simulink model "PMSM_FOC_Tractio"  (R2019b)
settings: Solver=FixedStepAuto  StartTime=0.0  StopTime=10  RelTol=1e-3
model workspace (MAT data in the model file):
  wc : Simulink.Parameter (value not decoded)
values from neighbouring files (symbols this model uses):
  Cosine_table = 1.0 0.99999529 0.99999058 0.99998587 0.99998116 0.99996704 0.99995291 0.99993885 0.99992472 0.99990118 0.99987763 0.99985409 0.9998306 0.99979764 0.99976468 0.99973178 0.99969882 0.99965644 0.99961412 0.99957174 0.99952942 0.99947762 0.99942589 0.99937415 0.99932235 0.9992612 0.99920005 0.99913889 0.99907768 0.99900717 0.99893659 0.99886602 0.99879545 0.99871546 0.99863547 0.99855554 0.99847555 0.    [Hall_HFI_FOC_Data.sldd]
  Flux = 0.00529276    [Hall_HFI_FOC_Data.sldd]
  MTPA_id_table = 0.22889 0.23462678 0.23770036 0.2381243 0.23591207 0.23107713 0.2236329 0.21359272 0.20096992 0.18577772 0.16802935 0.14773798 0.12491672 0.099578641 0.071736768 0.041404068 0.0085934745 -0.026682133 -0.064409919 -0.10457709 -0.14717092 -0.1921787 -0.2395878 -0.28938559 -0.34155953 -0.39609709 -0.45298585 -0.51221335 -0.57376724 -0.63763517 -0.70380485 -0.77226412 -0.84300071 -0.91600245 -0.991257    [Hall_HFI_FOC_Data.sldd]
  MTPA_iq_table = -1.0417 -0.16083497 0.71926296 1.5985928 2.4771533 3.3549435 4.2319627 5.1082091 5.9836826 6.8583813 7.732305 8.6054525 9.4778223 10.349415 11.220228 12.090261 12.959513 13.827983 14.69567 15.562573 16.428694 17.294027 18.158575 19.022335 19.885307 20.747492 21.608887 22.469492 23.329306 24.188328 25.046556 25.903992 26.760633 27.616482 28.471533 29.325788 30.179247 31.031908 31.883772 32.734837 3    [Hall_HFI_FOC_Data.sldd]
  MTPA_Te_Max = 800.0    [Hall_HFI_FOC_Data.sldd]
  MTPA_Te_Min = 0.0    [Hall_HFI_FOC_Data.sldd]
  Sine_table = 0.0 0.0015339879 0.0030679768 0.0046019657 0.0061359555 0.0076698866 0.0092038177 0.010737749 0.012271681 0.013805497 0.015339312 0.016873131 0.018406944 0.019940587 0.021474229 0.023007872 0.024541514 0.026074925 0.027608337 0.029141748 0.03067516 0.032208283 0.033741407 0.035274528 0.036807653 0.038340431 0.039873205 0.04140598 0.042938754 0.04447113 0.046003502 0.047535874 0.049068246 0.0506001    [Hall_HFI_FOC_Data.sldd]
undefined symbols (not defined in the file or in its folder): CL_Param, ctrlParamsPI, DiscIntNeverNeededParam, Flux_weak, HFI, inverter, magnitude, OPL_Param, pmsm, sigbuilder_block, SMO, SVPWM
libraries: powerlib x22, fl_lib x18, simulink x7, nesl_utility x7, powerlib_meascontrol x3, dspstat3 x3, powerlib_extras x1, ee_lib x1
(part 2 of 4)

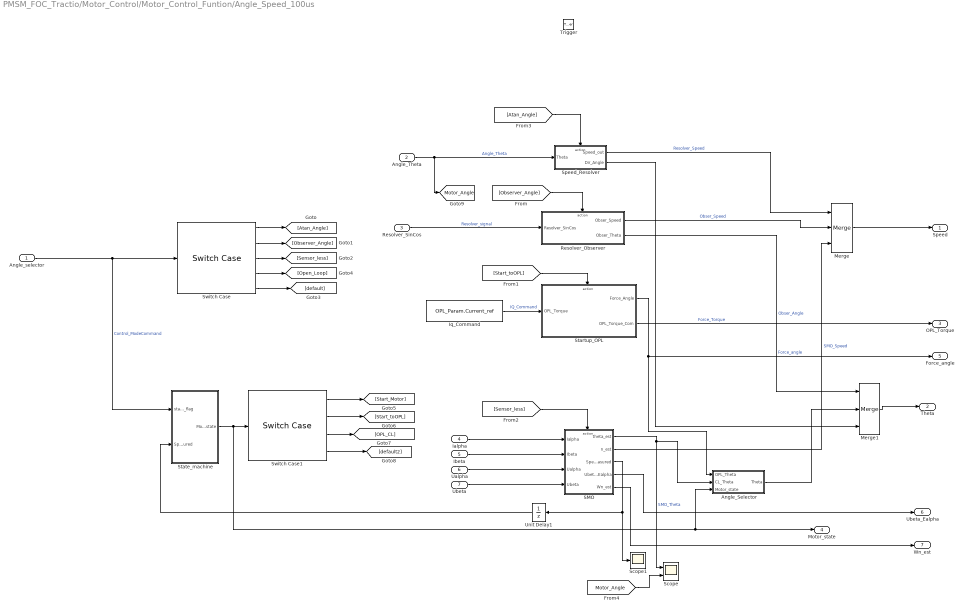
== system PMSM_FOC_Tractio/Motor_Control/Motor_Control_Funtion/Angle_Speed_100us ==
  Angle_selector : Inport
  Angle_Theta : Inport  Port=2  OutMin=0  OutMax=2*pi
  Resolver_SinCos : Inport  Port=3  OutMin=0  OutMax=2*pi
  Ialpha : Inport  Port=4
  Ibeta : Inport  Port=5
  Ualpha : Inport  Port=6
  Ubeta : Inport  Port=7
  Trigger : TriggerPort  TriggerType=function-call  VariantControl=Variant  SampleTimeType=periodic  SampleTime=-1  PortDimensions=1
  Angle_Selector : Subsystem  TreatAsAtomicUnit=on
      settings: RTWSystemCode=Nonreusable function  RTWFcnNameOpts=Use subsystem name
  Iq_Command : Constant  Value=OPL_Param.Current_ref  SampleTime=-1
  Merge : Merge  Inputs=3
  Merge1 : Merge  Inputs=3
  Resolver_Observer : Subsystem
      settings: RTWSystemCode=Nonreusable function  RTWFcnNameOpts=Use subsystem name
  SMO : Subsystem  TreatAsAtomicUnit=on
      settings: RTWSystemCode=Nonreusable function  RTWFcnNameOpts=Use subsystem name
  Scope : Scope  NumInputPorts=2
  Scope1 : Scope
  Speed_Resolver : Subsystem  TreatAsAtomicUnit=on
      settings: RTWSystemCode=Nonreusable function  RTWFcnNameOpts=Use subsystem name
  Startup_OPL : Subsystem  TreatAsAtomicUnit=on  SystemSampleTime=inverter.Ts
      settings: RTWSystemCode=Nonreusable function  RTWFcnNameOpts=Use subsystem name
  State_machine : Stateflow chart  BlockKeywords=__PRM__SERIALIZED__DATA__:Stateflow Chart,Stateflow Diagram  TreatAsAtomicUnit=on
      settings: RTWSystemCode=Nonreusable function  RTWFcnNameOpts=Use subsystem name
  Switch Case : SwitchCase  CaseConditions={1,2,3,4}
  Switch Case1 : SwitchCase  CaseConditions={1,2,3}
  Unit Delay1 : UnitDelay  SampleTime=-1  HasFrameUpgradeWarning=on
  Speed : Outport
  Theta : Outport  Port=2
  OPL_Torque : Outport  Port=3
  Motor_state : Outport  Port=4
  Force_angle : Outport  Port=5
  Ubeta_Ealpha : Outport  Port=6
  Wn_est : Outport  Port=7
  tag scope: Motor_Angle=global
  wires:
  [Start_toOPL] -> Startup_OPL/Action
  [Sensor_less] -> SMO/Action
  Resolver_SinCos/1 -> Resolver_Observer/1(Resolver_SinCos)  "Resolver_signal"
  [Observer_Angle] -> Resolver_Observer/Action
  Iq_Command/1 -> Startup_OPL/1(OPL_Torque)  "IQ_Command"
  Resolver_Observer/2(Obser_Theta) -> Merge1/1  "Obser_Angle"
  Ialpha/1 -> SMO/1(Ialpha)
  Ibeta/1 -> SMO/2(Ibeta)
  Ualpha/1 -> SMO/3(Ualpha)
  Ubeta/1 -> SMO/4(Ubeta)
  Merge/1 -> Speed/1
  Merge1/1 -> Theta/1
  Angle_selector/1 -> State_machine/1(start_flag), Switch Case/1  "Control_ModeCommand"
  Switch Case/5 -> [default]
  Switch Case/3 -> [Sensor_less]
  Switch Case/1 -> [Atan_Angle]
  Switch Case/4 -> [Open_Loop]
  Switch Case/2 -> [Observer_Angle]
  Speed_Resolver/1(Speed_out) -> Merge/1  "Resolver_Speed"
  Angle_Theta/1 -> [Motor_Angle], Speed_Resolver/1(Theta)  "Angle_Theta"
  [Atan_Angle] -> Speed_Resolver/Action
  SMO/2(n_est) -> Merge/3  "SMO_Speed"
  Resolver_Observer/1(Obser_Speed) -> Merge/2  "Obser_Speed"
  Startup_OPL/2(OPL_Torque_Com) -> OPL_Torque/1  "Force_Torque"
  Speed_Resolver/2(Dir_Angle) -> Merge1/3
  Switch Case1/3 -> [OPL_CL]
  Switch Case1/2 -> [Start_toOPL]
  Switch Case1/1 -> [Start_Motor]
  Switch Case1/4 -> [default2]
  State_machine/1(Motor_state) -> Angle_Selector/3(Motor_state), Motor_state/1, Switch Case1/1
  Unit Delay1/1 -> State_machine/2(Speed_Measured)
  SMO/1(theta_est) -> Scope/1, Angle_Selector/2(CL_Theta)  "SMO_Theta"
  Startup_OPL/1(Force_Angle) -> Angle_Selector/1(OPL_Theta), Force_angle/1  "Force_angle"
  Angle_Selector/1(Theta) -> Merge1/2
  [Motor_Angle] -> Scope/2
  SMO/3(Speed_Measured) -> Unit Delay1/1, Scope1/1
  SMO/4(Ubeta_Ealpha) -> Ubeta_Ealpha/1
  SMO/5(Wn_est) -> Wn_est/1

== system PMSM_FOC_Tractio/Motor_Control/Motor_Control_Funtion/Control_Command_2ms ==
  Control_Mode : Inport
  Speed_target : Inport  Port=2
  Speed_Mesured : Inport  Port=3  OutMin=0  OutMax=2*pi
  HFI_State : Inport  Port=4
  Trigger : TriggerPort  TriggerType=function-call  VariantControl=Variant  SampleTimeType=periodic  SampleTime=-1  PortDimensions=1
  IQ_Command : Constant  Value=CL_Param.Current_IQref  OutDataTypeStr=single  SampleTime=-1
  Merge : Merge
  Speed_PI : Subsystem  TreatAsAtomicUnit=on  SystemSampleTime=inverter.Ts
      settings: RTWSystemCode=Nonreusable function
  Switch Case : SwitchCase  CaseConditions={1,2}
  Switch Case Action Subsystem : Subsystem  TreatAsAtomicUnit=on
      settings: RTWSystemCode=Nonreusable function
  Te_ref : Outport
  wires:
  Switch Case Action Subsystem/1(Iq_out) -> Merge/2
  IQ_Command/1 -> Switch Case Action Subsystem/1(Iq_in)  "IQ_Command"
  Switch Case/3 -> [default]
  [Torque_Mode] -> Switch Case Action Subsystem/Action
  Switch Case/2 -> [Torque_Mode]
  Switch Case/1 -> [Speed_Mode]
  Control_Mode/1 -> Switch Case/1  "Control_ModeCommand"
  [Speed_Mode] -> Speed_PI/Action
  Speed_PI/1(Iq_ref) -> Merge/1  "Iq_ref"
  Merge/1 -> Te_ref/1
  Speed_target/1 -> Speed_PI/1(Speed_Command)  "Speed_target"
  Speed_Mesured/1 -> Speed_PI/2(Speed_Measured)  "Speed_Measured"
  HFI_State/1 -> Speed_PI/3(HFI_State)  "Control_ModeCommand"

== system PMSM_FOC_Tractio/Motor_Control/Motor_Control_Funtion/FOC_Control_100us ==
  Phase_CurrentABC : Inport  PortDimensions=3
  Angle_Theta : Inport  Port=2  OutMin=0  OutMax=2*pi
  Te_ref : Inport  Port=3
  Motor_state : Inport  Port=4
  OPL_Iq : Inport  Port=5
  Trigger : TriggerPort  TriggerType=function-call  VariantControl=Variant  SampleTimeType=periodic  SampleTime=-1  PortDimensions=1
  FOC : Subsystem  TreatAsAtomicUnit=on
      settings: RTWSystemCode=Nonreusable function  RTWFcnNameOpts=Use subsystem name
  Iq_selector : Subsystem  TreatAsAtomicUnit=on
      settings: RTWSystemCode=Nonreusable function  RTWFcnNameOpts=Use subsystem name
  MTPA : Subsystem  TreatAsAtomicUnit=on
      settings: RTWSystemCode=Nonreusable function  RTWFcnNameOpts=Use subsystem name
  Ta : Outport
  Tb : Outport  Port=2
  Tc : Outport  Port=3
  Ialpha : Outport  Port=4
  Ibeta : Outport  Port=5
  Valpha : Outport  Port=6
  Vbeta : Outport  Port=7
  Id : Outport  Port=8
  Iq : Outport  Port=9
  HFI_Theta : Outport  Port=10
  RUN_State : Outport  Port=11
  HFI_Speed : Outport  Port=12
  wires:
  FOC/1(Ta) -> Ta/1  "Ta"
  FOC/2(Tb) -> Tb/1  "Tb"
  FOC/3(Tc) -> Tc/1  "Tc"
  Angle_Theta/1 -> FOC/3(Angle_Theta)  "Angle_Theta"
  FOC/4(Ialpha) -> Ialpha/1  "Ialpha"
  FOC/5(Ibeta) -> Ibeta/1  "Ibeta"
  FOC/6(Valpha) -> Valpha/1  "V_alpha"
  FOC/7(Vbeta) -> Vbeta/1  "V_beta"
  FOC/8(Id) -> Id/1  "Id_measured"
  FOC/9(Iq) -> Iq/1  "Iq_measured"
  Phase_CurrentABC/1 -> FOC/4(Phase_CurrentABC)  "Phase_CurrentABC"
  FOC/11(HFI_Theta) -> HFI_Theta/1  "HFI_Theta"
  FOC/10(RUN_State) -> RUN_State/1
  FOC/12(HFI_Speed) -> HFI_Speed/1
  MTPA/1(Id_ref) -> FOC/1(Id_target)  "Id_ref"
  MTPA/2(Iq_ref) -> Iq_selector/2(PI_IQ)  "Iq_ref"
  Iq_selector/1(Iq_ref) -> FOC/2(Iq_target)
  Te_ref/1 -> MTPA/1(Te_ref)
  Motor_state/1 -> Iq_selector/1(Motor_state)
  OPL_Iq/1 -> Iq_selector/3(OPL_IQ)

== system PMSM_FOC_Tractio/PMSM/Resolver/Meas Vxy ==
  Electrical Reference{1..4} (4 alike) : fl_lib/Electrical/Electrical Elements/Electrical Reference
  PS-Simulink Converter : nesl_utility/PS-Simulink Converter  PhysicalDomain=network_engine_domain  SubClassName=ps_output  LeftPortType=input  RightPortType=output  PseudoPeriodic=off  Frequencies=[]  Unit=1  AffineConversion=off
  PS-Simulink Converter1 : nesl_utility/PS-Simulink Converter  PhysicalDomain=network_engine_domain  SubClassName=ps_output  LeftPortType=input  RightPortType=output  PseudoPeriodic=off  Frequencies=[]  Unit=1  AffineConversion=off
  Resistor : fl_lib/Electrical/Electrical Elements/Resistor  R=1e3 Ohm  i_specify=off  i_priority=None  i=0 A  i_nominal_specify=off  i_nominal_unit=A  i_nominal_value=1  v_specify=off  v_priority=None  v=0 V  v_nominal_specify=off  v_nominal_unit=V  v_nominal_value=1
  Resistor1 : fl_lib/Electrical/Electrical Elements/Resistor  R=1e3 Ohm  i_specify=off  i_priority=None  i=0 A  i_nominal_specify=off  i_nominal_unit=A  i_nominal_value=1  v_specify=off  v_priority=None  v=0 V  v_nominal_specify=off  v_nominal_unit=V  v_nominal_value=1
  VS1 : fl_lib/Electrical/Electrical Sensors/Voltage Sensor
  VS2 : fl_lib/Electrical/Electrical Sensors/Voltage Sensor
  x1 : PMIOPort  Side=Left
  x2 : PMIOPort  Port=2  Side=Left
  y1 : PMIOPort  Port=3  Side=Left
  y2 : PMIOPort  Port=4  Side=Left
  Vx : Outport  VectorParamsAs1DForOutWhenUnconnected=off
  Vy : Outport  Port=2  VectorParamsAs1DForOutWhenUnconnected=off
  wires:
  PS-Simulink Converter1/1 -> Vy/1
  PS-Simulink Converter/1 -> Vx/1
  connections:
  VS1/RConn1 -- PS-Simulink Converter/LConn1
  Resistor/RConn1 -- x2/RConn1 -- Electrical Reference2/LConn1
  Electrical Reference1/LConn1 -- VS1/RConn2
  y2/RConn1 -- Electrical Reference4/LConn1 -- Resistor1/RConn1
  VS2/LConn1 -- y1/RConn1 -- Resistor1/LConn1
  Electrical Reference3/LConn1 -- VS2/RConn2
  VS2/RConn1 -- PS-Simulink Converter1/LConn1
  Resistor/LConn1 -- x1/RConn1 -- VS1/LConn1

== system PMSM_FOC_Tractio/PMSM/Resolver/Vp ==
  Electrical Reference1 : fl_lib/Electrical/Electrical Elements/Electrical Reference
  PS-Simulink Converter2 : nesl_utility/PS-Simulink Converter  PhysicalDomain=network_engine_domain  SubClassName=ps_output  LeftPortType=input  RightPortType=output  PseudoPeriodic=off  Frequencies=[]  Unit=1  AffineConversion=off
  VS1 : fl_lib/Electrical/Electrical Sensors/Voltage Sensor
  Vp1 : fl_lib/Electrical/Electrical Sources/AC Voltage Source  amp=5 V  shift=0 rad  frequency=1e4 Hz  omega=0 rad/s
  p1 : PMIOPort  Side=Right
  p2 : PMIOPort  Port=2  Side=Right
  Vp : Outport  VectorParamsAs1DForOutWhenUnconnected=off
  wires:
  PS-Simulink Converter2/1 -> Vp/1
  connections:
  VS1/RConn1 -- PS-Simulink Converter2/LConn1
  Electrical Reference1/LConn1 -- p2/RConn1 -- VS1/RConn2 -- Vp1/RConn1
  VS1/LConn1 -- Vp1/LConn1 -- p1/RConn1

== system PMSM_FOC_Tractio/PMSM/Resolver_SinCos/If Action Subsystem ==
  In1 : Inport
  Action Port : ActionPort  ActionPortLabel=if(u1 == 1)
  Out1 : Outport
  wires:
  In1/1 -> Out1/1

== system PMSM_FOC_Tractio/PMSM/Resolver_SinCos/If Action Subsystem1 ==
  In1 : Inport
  Action Port : ActionPort  ActionPortLabel=else
  Gain : Gain  Gain=-1
  Out1 : Outport
  wires:
  In1/1 -> Gain/1
  Gain/1 -> Out1/1

== system PMSM_FOC_Tractio/PMSM/Resolver_SinCos/If Action Subsystem2 ==
  In1 : Inport
  Action Port : ActionPort  ActionPortLabel=if(u1 == 1)
  Out1 : Outport
  wires:
  In1/1 -> Out1/1

== system PMSM_FOC_Tractio/PMSM/Resolver_SinCos/If Action Subsystem3 ==
  In1 : Inport
  Action Port : ActionPort  ActionPortLabel=else
  Gain : Gain  Gain=-1
  Out1 : Outport
  wires:
  In1/1 -> Gain/1
  Gain/1 -> Out1/1

== system PMSM_FOC_Tractio/PMSM/Resolver_SinCos/Subsystem ==
  In1 : Inport
  Trigger : TriggerPort  VariantControl=Variant  SampleTimeType=periodic  SampleTime=-1  PortDimensions=1
  Out1 : Outport
  wires:
  In1/1 -> Out1/1

== system PMSM_FOC_Tractio/PMSM/Resolver_SinCos/Subsystem1 ==
  In1 : Inport
  Trigger : TriggerPort  VariantControl=Variant  SampleTimeType=periodic  SampleTime=-1  PortDimensions=1
  Out1 : Outport
  wires:
  In1/1 -> Out1/1

== system PMSM_FOC_Tractio/PMSM/Resolver_SinCos/Subsystem2 ==
  Trigger : TriggerPort  VariantControl=Variant  SampleTimeType=periodic  SampleTime=-1  PortDimensions=1
  Add : Sum
  Constant : Constant
  Constant1 : Constant  Value=2
  Memory : Memory  InheritSampleTime=on
  Mod : Math  Operator=mod  SignedPower=off  SaturateOnIntegerOverflow=on
  Out1 : Outport
  wires:
  Add/1 -> Mod/1, Memory/1
  Constant/1 -> Add/1
  Memory/1 -> Add/2
  Mod/1 -> Out1/1  "Theta"
  Constant1/1 -> Mod/2

== system PMSM_FOC_Tractio/PMSM/Resolver_SinCos/Subsystem3 ==
  Trigger : TriggerPort  VariantControl=Variant  SampleTimeType=periodic  SampleTime=-1  PortDimensions=1
  Add : Sum
  Constant : Constant
  Constant1 : Constant  Value=2
  Memory : Memory  InheritSampleTime=on
  Mod : Math  Operator=mod  SignedPower=off  SaturateOnIntegerOverflow=on
  Out1 : Outport
  wires:
  Add/1 -> Mod/1, Memory/1
  Constant/1 -> Add/1
  Memory/1 -> Add/2
  Mod/1 -> Out1/1  "Theta"
  Constant1/1 -> Mod/2

== system PMSM_FOC_Tractio/PMSM/W_R/Torque Sensor ==
  Ideal Torque Sensor : fl_lib/Mechanical/Mechanical Sensors/Ideal Torque Sensor
  PS-Simulink Converter : nesl_utility/PS-Simulink Converter  PhysicalDomain=network_engine_domain  SubClassName=ps_output  LeftPortType=input  RightPortType=output  PseudoPeriodic=off  Frequencies=[]  Unit=N*m  AffineConversion=off
  R : PMIOPort  Side=Right
  C : PMIOPort  Port=2  Side=Left
  tag scope: trqDynoOC=global
  wires:
  PS-Simulink Converter/1 -> [trqDynoOC]
  connections:
  PS-Simulink Converter/LConn1 -- Ideal Torque Sensor/RConn2
  R/RConn1 -- Ideal Torque Sensor/LConn1
  Ideal Torque Sensor/RConn1 -- C/RConn1

== system PMSM_FOC_Tractio/Motor_Control/Motor_Control_Funtion/Angle_Speed_100us/Angle_Selector ==
  OPL_Theta : Inport
  CL_Theta : Inport  Port=2
  Motor_state : Inport  Port=3
  If1 : If  IfExpression=u1 ==2  ElseIfExpressions=u1 ==3  ShowElse=off
  Merge : Merge
  Scope : Scope  NumInputPorts=2
  Subsystem : Subsystem
  Subsystem1 : Subsystem
  Theta : Outport
  wires:
  Motor_state/1 -> If1/1
  If1/1 -> Subsystem/Action
  OPL_Theta/1 -> Scope/1, Subsystem/1(In1)
  CL_Theta/1 -> Scope/2, Subsystem1/1(In1)
  Subsystem/1(Out1) -> Merge/1
  Subsystem1/1(Out1) -> Merge/2
  Merge/1 -> Theta/1  "FOC_Angle"
  If1/2 -> Subsystem1/Action

== system PMSM_FOC_Tractio/Motor_Control/Motor_Control_Funtion/Angle_Speed_100us/Resolver_Observer ==
  Resolver_SinCos : Inport
  Action Port : ActionPort  ActionPortLabel=case [ 2 ]:
  Angle_calibration : Subsystem  TreatAsAtomicUnit=on
      settings: RTWSystemCode=Nonreusable function  RTWFcnNameOpts=Use subsystem name
  Resolver_Angle_cacl : Subsystem  TreatAsAtomicUnit=on
      settings: RTWSystemCode=Nonreusable function  RTWFcnNameOpts=Use subsystem name  RTWFileNameOpts=Use subsystem name  FunctionInterfaceSpec=Allow arguments
  Scope : Scope
  Scope1 : Scope
  Obser_Speed : Outport
  Obser_Theta : Outport  Port=2
  wires:
  Resolver_Angle_cacl/1(Velocity) -> Scope/1, Obser_Speed/1  "Obser_Speed"
  Resolver_Angle_cacl/2(Angle) -> Angle_calibration/1(Angle_input)
  Resolver_SinCos/1 -> Resolver_Angle_cacl/1(Sin_Cos)
  Angle_calibration/1(Angle_output) -> Scope1/1, Obser_Theta/1  "Obser_Angle"

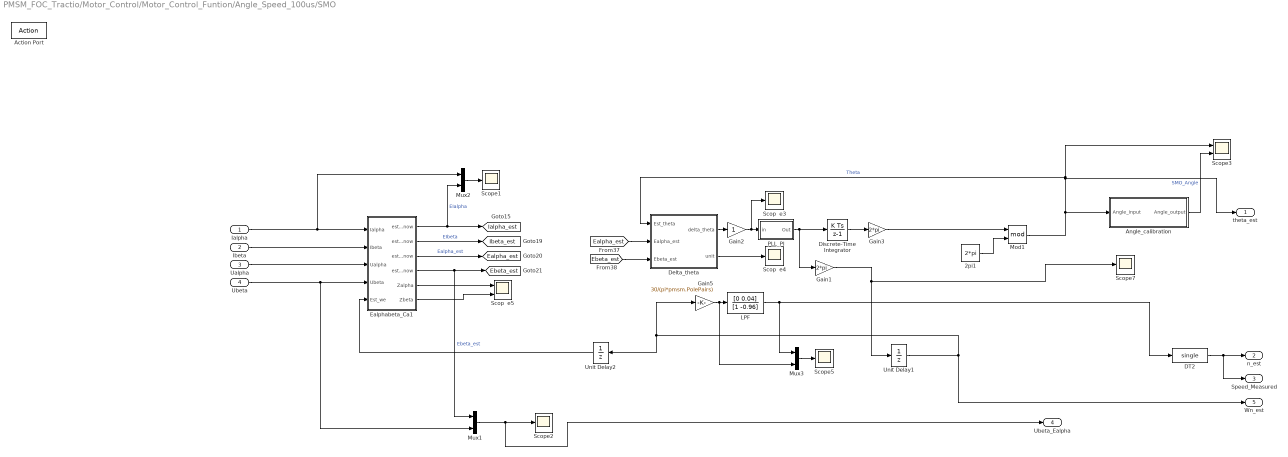
== system PMSM_FOC_Tractio/Motor_Control/Motor_Control_Funtion/Angle_Speed_100us/SMO ==
  Ialpha : Inport
  Ibeta : Inport  Port=2
  Ualpha : Inport  Port=3
  Ubeta : Inport  Port=4
  Action Port : ActionPort  ActionPortLabel=case [ 3 ]:
  2pi1 : Constant  Value=2*pi  OutDataTypeStr=single
  Angle_calibration : Subsystem  TreatAsAtomicUnit=on
      settings: RTWSystemCode=Nonreusable function  RTWFcnNameOpts=Use subsystem name
  DT2 : DataTypeConversion  OutDataTypeStr=single
  Delta_theta : Subsystem  TreatAsAtomicUnit=on
      settings: RTWSystemCode=Nonreusable function  RTWFcnNameOpts=Use subsystem name
  Discrete-Time Integrator : DiscreteIntegrator  SampleTime=-1  ICPrevOutput=DiscIntNeverNeededParam  ICPrevScaledInput=DiscIntNeverNeededParam
  Ealphabeta_Ca1 : Subsystem  TreatAsAtomicUnit=on
      settings: RTWSystemCode=Nonreusable function  RTWFcnNameOpts=Use subsystem name
  Gain1 : Gain  Gain=2*pi
  Gain2 : Gain
  Gain3 : Gain  Gain=2*pi  OutDataTypeStr=single
  Gain5 : Gain  Gain=30/(pi*pmsm.PolePairs)
  LPF : DiscreteFilter  Numerator=[0 0.04]  Denominator=[1 -0.96]  SampleTime=inverter.Ts
  Mod1 : Math  Operator=mod  SignedPower=off  SaturateOnIntegerOverflow=on
  Mux1 : Mux  Inputs=2
  Mux2 : Mux  Inputs=2
  Mux3 : Mux  Inputs=2
  PLL_PI : Subsystem  mask{kp=SMO.PLL_KP, ki=SMO.PLL_Ki, Ts=inverter.Ts}
  Scop  e3 : Scope
  Scop  e4 : Scope
  Scop  e5 : Scope  NumInputPorts=2
  Scope{1..2,5,7} (4 alike) : Scope
  Scope3 : Scope  NumInputPorts=2
  Unit Delay1 : UnitDelay  SampleTime=-1  HasFrameUpgradeWarning=on
  Unit Delay2 : UnitDelay  SampleTime=-1  HasFrameUpgradeWarning=on
  theta_est : Outport
  n_est : Outport  Port=2
  Speed_Measured : Outport  Port=3
  Ubeta_Ealpha : Outport  Port=4
  Wn_est : Outport  Port=5
  tag scope: Ealpha_est=global, Ebeta_est=global, Ialpha_est=global, Ibeta_est=global
  wires:
  Ualpha/1 -> Ealphabeta_Ca1/3(Ualpha)
  Ealphabeta_Ca1/3(est_ealpha_now) -> [Ealpha_est]  "Ealpha_est"
  Ialpha/1 -> Ealphabeta_Ca1/1(Ialpha), Mux2/1
  Ibeta/1 -> Ealphabeta_Ca1/2(Ibeta)
  Ubeta/1 -> Ealphabeta_Ca1/4(Ubeta), Mux1/2
  Ealphabeta_Ca1/6(Zbeta) -> Scop  e5/2
  Ealphabeta_Ca1/1(est_Ialpha_now) -> Mux2/2, [Ialpha_est]  "EIalpha"
  Mux1/1 -> Ubeta_Ealpha/1, Scope2/1
  Ealphabeta_Ca1/4(est_ebeta_now) -> [Ebeta_est], Mux1/1  "Ebeta_est"
  Ealphabeta_Ca1/5(Zalpha) -> Scop  e5/1
  Ealphabeta_Ca1/2(est_Ibeta_now) -> [Ibeta_est]  "EIbeta"
  Mux2/1 -> Scope1/1
  LPF/1 -> Mux3/1, DT2/1
  [Ebeta_est] -> Delta_theta/3(Ebeta_est)
  Delta_theta/1(delta_theta) -> Gain2/1
  Unit Delay1/1 -> Gain5/1, Unit Delay2/1, Wn_est/1
  Gain2/1 -> Scop  e3/1, PLL_PI/1(in)
  Gain3/1 -> Mod1/1
  [Ealpha_est] -> Delta_theta/2(Ealpha_est)
  Discrete-Time Integrator/1 -> Gain3/1
  Mod1/1 -> Scope3/1, Delta_theta/1(Est_theta), theta_est/1, Angle_calibration/1(Angle_input)  "Theta"
  PLL_PI/1(Out) -> Discrete-Time Integrator/1, Gain1/1
  2pi1/1 -> Mod1/2
  Gain1/1 -> Unit Delay1/1, Scope7/1
  Mux3/1 -> Scope5/1
  Delta_theta/2(unit) -> Scop  e4/1
  Gain5/1 -> Mux3/2, LPF/1
  Unit Delay2/1 -> Ealphabeta_Ca1/5(Est_we)
  DT2/1 -> Speed_Measured/1, n_est/1
  Angle_calibration/1(Angle_output) -> Scope3/2  "SMO_Angle"

== system PMSM_FOC_Tractio/Motor_Control/Motor_Control_Funtion/Angle_Speed_100us/Speed_Resolver ==
  Theta : Inport
  Action Port : ActionPort  ActionPortLabel=case [ 1 ]:
  DT2 : DataTypeConversion  OutDataTypeStr=single
  Scope : Scope
  Scope1 : Scope
  Speed_cacl : Subsystem  TreatAsAtomicUnit=on
      settings: RTWSystemCode=Nonreusable function  RTWFcnNameOpts=Use subsystem name
  Speed_out : Outport
  Dir_Angle : Outport  Port=2
  wires:
  Theta/1 -> DT2/1, Speed_cacl/1(position)  "Theta_input"
  Speed_cacl/1(Speed_RPM) -> Scope1/1, Speed_out/1  "Speed_RPM_Filtered"
  DT2/1 -> Scope/1, Dir_Angle/1  "Direct_Angle"

== system PMSM_FOC_Tractio/Motor_Control/Motor_Control_Funtion/Angle_Speed_100us/Startup_OPL ==
  OPL_Torque : Inport
  Action Port : ActionPort  ActionPortLabel=case [ 2 ]:
  2pi1 : Constant  Value=2*pi  OutDataTypeStr=single
  Add : Sum
  Constant : Constant  Value=OPL_Param.Constant
  DT1 : DataTypeConversion  OutDataTypeStr=single
  DT2 : DataTypeConversion  OutDataTypeStr=single
  Discrete-Time Integrator : DiscreteIntegrator  SampleTime=-1  ICPrevOutput=DiscIntNeverNeededParam  ICPrevScaledInput=DiscIntNeverNeededParam
  Gain2 : Gain  Gain=pmsm.PolePairs*2*pi/60  OutDataTypeStr=single  ParamDataTypeStr=Inherit: Same as input
  Memory : Memory  InheritSampleTime=on
  Mod1 : Math  Operator=mod  SignedPower=off  SaturateOnIntegerOverflow=on
  Saturation : Saturate  UpperLimit=OPL_Param.Target_RPMMax  LowerLimit=OPL_Param.Target_RPMMin
  Scope : Scope
  Scope1 : Scope
  Scope2 : Scope
  Force_Angle : Outport
  OPL_Torque_Com : Outport  Port=2
  wires:
  Gain2/1 -> Discrete-Time Integrator/1  "Speed"
  Discrete-Time Integrator/1 -> Mod1/1
  2pi1/1 -> Mod1/2
  OPL_Torque/1 -> DT2/1
  Constant/1 -> Scope2/1, Add/1
  Add/1 -> Saturation/1, Memory/1
  Memory/1 -> Add/2
  Saturation/1 -> Gain2/1
  Mod1/1 -> DT1/1  "Theta"
  DT1/1 -> Scope/1, Force_Angle/1  "Force_Angle"
  DT2/1 -> Scope1/1, OPL_Torque_Com/1

== system PMSM_FOC_Tractio/Motor_Control/Motor_Control_Funtion/Control_Command_2ms/Speed_PI ==
  Speed_Command : Inport
  Speed_Measured : Inport  Port=2
  HFI_State : Inport  Port=3
  Action Port : ActionPort  ActionPortLabel=case [ 1 ]:
  Add2 : Sum  Inputs=|+-
  Scope2 : Scope
  Speed_PI : Subsystem
  Iq_ref : Outport  VectorParamsAs1DForOutWhenUnconnected=off
  wires:
  Speed_Command/1 -> Add2/1
  Speed_Measured/1 -> Add2/2
  Add2/1 -> Speed_PI/1(PI_input)  "currentControlError"
  Speed_PI/1(PI_out) -> Iq_ref/1, Scope2/1
  HFI_State/1 -> Speed_PI/2(HFI_State)

== system PMSM_FOC_Tractio/Motor_Control/Motor_Control_Funtion/Control_Command_2ms/Switch Case Action Subsystem ==
  Iq_in : Inport
  Action Port : ActionPort  ActionPortLabel=case [ 2 ]:
  Iq_out : Outport
  wires:
  Iq_in/1 -> Iq_out/1

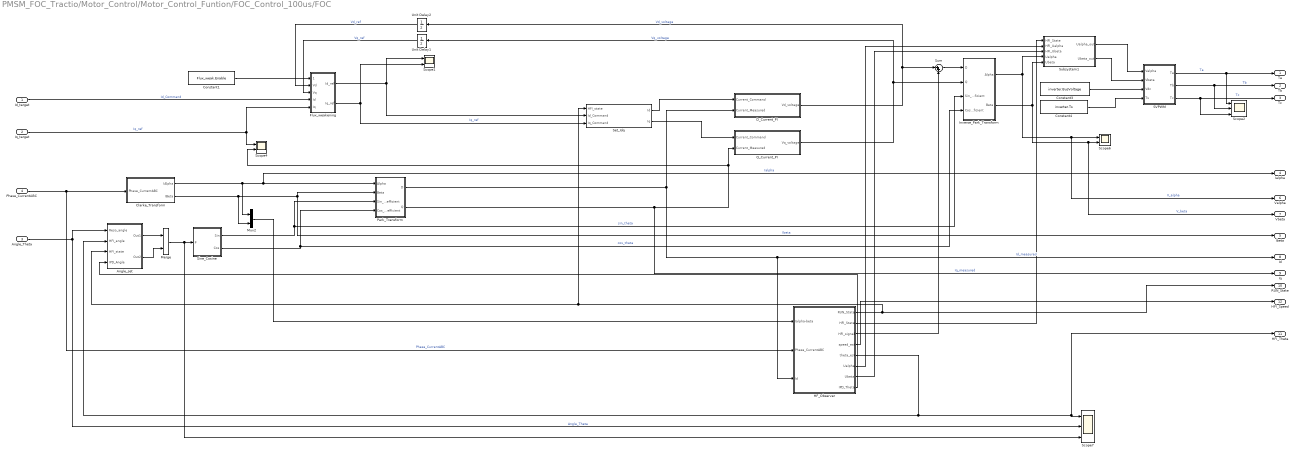
== system PMSM_FOC_Tractio/Motor_Control/Motor_Control_Funtion/FOC_Control_100us/FOC ==
  Id_target : Inport
  Iq_target : Inport  Port=2
  Angle_Theta : Inport  Port=3  OutMin=0  OutMax=2*pi
  Phase_CurrentABC : Inport  Port=4  PortDimensions=3
  Angle_set : Subsystem  TreatAsAtomicUnit=on
      settings: RTWSystemCode=Nonreusable function  RTWFcnNameOpts=Use subsystem name
  Clarke_Transform : Subsystem  TreatAsAtomicUnit=on
      settings: RTWSystemCode=Nonreusable function  RTWFcnNameOpts=Use subsystem name
  Constant1 : Constant  Value=Flux_weak.Enable  OutDataTypeStr=single
  Constant3 : Constant  Value=inverter.BusVoltage  OutDataTypeStr=single
  Constant4 : Constant  Value=inverter.Ts  OutDataTypeStr=single
  D_Current_PI : Subsystem  TreatAsAtomicUnit=on
      settings: RTWSystemCode=Nonreusable function  RTWFcnNameOpts=Use subsystem name
  "Flux_weakening " : Subsystem
  HF_Observer : Subsystem  TreatAsAtomicUnit=on
      settings: RTWSystemCode=Nonreusable function  RTWFcnNameOpts=Use subsystem name  RTWFileNameOpts=Use subsystem name
  Inverse_Park_Transform : Subsystem  TreatAsAtomicUnit=on
      settings: RTWSystemCode=Nonreusable function  RTWFcnNameOpts=Use subsystem name
      mask Display:
      | port_label('input',1,'D')
      | port_label('input',2,'Q')
      | port_label('input',3,'Sin')
      | port_label('input',4,'Cos')
      | port_label('output',1,'\alpha','texmode', 'on')
      | port_label('output',2,'\beta','texmode', 'on')
  Merge : Merge
  Mux2 : Mux  Inputs=2
  Park_Transform : Subsystem  TreatAsAtomicUnit=on
      settings: RTWSystemCode=Nonreusable function  RTWFcnNameOpts=Use subsystem name
      mask Display:
      | port_label('input',1,'\alpha','texmode', 'on')
      | port_label('input',2,'\beta','texmode', 'on')
      | port_label('input',3,'Sin')
      | port_label('input',4,'Cos')
      | port_label('output',1,'D')
      | port_label('output',2,'Q')
  Q_Current_PI : Subsystem  TreatAsAtomicUnit=on
      settings: RTWSystemCode=Nonreusable function  RTWFcnNameOpts=Use subsystem name
  SVPWM : Subsystem  AncestorBlock=SVPWM/SVPWM  TreatAsAtomicUnit=on  RTWFcnName=SVPWM  RTWFileName=SVPWM
      settings: RTWSystemCode=Nonreusable function  RTWFcnNameOpts=Use subsystem name
      mask Display:
      | plot([0.000 0.020 0.041 0.061 0.082 0.102 0.122 0.143 0.163 0.184 0.204 0.224 0.245 0.265 0.286 0.306 0.327 0.347 0.367 0.388 0.408 0.429 0.449 0.469 0.490 0.510 0.531 0.551 0.571 0.592 0.612 0.633 0.653 0.673 0.694 0.714 0.735 0.755 0.776 0.796 0.816 0.837 0.857 0.878 0.898 0.918 0.939 0.959 0.980 1.000 ], ...
      |      [0.500 0.586 0.671 0.753 0.831 0.858 0.875 0.885 0.890 0.887 0.879 0.864 0.844 0.855 0.872 0.884 0.889 0.888 0.881 0.867 0.847 0.793 0.713 0.629 0.543 0.457 0.371 0.287 0.207 0.153 0.133 0.119 0.112 0.111 0.116 0.128 0.145 0.156 0.136 0.121 0.113 0.110 0.115 0.125 0.142 0.169 0.247 0.329 0.414 0.500 ])
  Scope1 : Scope  NumInputPorts=2
  Scope2 : Scope  NumInputPorts=3
  Scope4 : Scope  NumInputPorts=2
  Scope6 : Scope  NumInputPorts=2
  Scope7 : Scope  NumInputPorts=3
  Set_Idq : Subsystem  TreatAsAtomicUnit=on
      settings: RTWSystemCode=Nonreusable function  RTWFcnNameOpts=Use subsystem name
  Sine_Cosine : Subsystem  TreatAsAtomicUnit=on
      settings: RTWSystemCode=Nonreusable function  RTWFcnNameOpts=Use subsystem name
  Subsystem1 : Subsystem
  Sum : Sum  Inputs=|++
  Unit Delay1 : UnitDelay  SampleTime=-1  HasFrameUpgradeWarning=on
  Unit Delay2 : UnitDelay  SampleTime=-1  HasFrameUpgradeWarning=on
  Ta : Outport
  Tb : Outport  Port=2
  Tc : Outport  Port=3
  Ialpha : Outport  Port=4
  Ibeta : Outport  Port=5
  Valpha : Outport  Port=6
  Vbeta : Outport  Port=7
  Id : Outport  Port=8
  Iq : Outport  Port=9
  RUN_State : Outport  Port=10
  HFI_Theta : Outport  Port=11
  HFI_Speed : Outport  Port=12
  wires:
  Park_Transform/1(D) -> Id/1, HF_Observer/3(Id), D_Current_PI/2(Current_Measured)  "Id_measured"
  Constant4/1 -> SVPWM/4(Ts)
  SVPWM/3(Tc) -> Tc/1, Scope2/3  "Tc"
  SVPWM/2(Tb) -> Scope2/2, Tb/1  "Tb"
  Park_Transform/2(Q) -> Iq/1, Scope4/2, Q_Current_PI/2(Current_Measured)  "Iq_measured"
  Sine_Cosine/2(Cos) -> Park_Transform/4(Cos_Coefficient), Inverse_Park_Transform/4(Cos_Coefficient)  "cos_theta"
  Sine_Cosine/1(Sin) -> Park_Transform/3(Sin_Coefficient), Inverse_Park_Transform/3(Sin_Coefficient)  "sin_theta"
  Constant3/1 -> SVPWM/3(Vdc)
  D_Current_PI/1(Vd_voltage) -> Unit Delay2/1, Sum/1  "Vd_voltage"
  Q_Current_PI/1(Vq_voltage) -> Unit Delay1/1, Inverse_Park_Transform/2(Q)  "Vq_voltage"
  SVPWM/1(Ta) -> Scope2/1, Ta/1  "Ta"
  Id_target/1 -> "Flux_weakening "/4(Id)  "Id_Command"
  Iq_target/1 -> "Flux_weakening "/5(Iq), Scope4/1  "Iq_ref"
  Clarke_Transform/2(IBeta) -> Mux2/2, Ibeta/1, Park_Transform/2(Beta)  "Ibeta"
  Clarke_Transform/1(IAlpha) -> Ialpha/1, Park_Transform/1(Alpha), Mux2/1  "Ialpha"
  Unit Delay2/1 -> "Flux_weakening "/2(Vd)  "Vd_ref"
  Unit Delay1/1 -> "Flux_weakening "/3(Vq)  "Vq_ref"
  "Flux_weakening "/1(Id_ref) -> Scope1/1, Set_Idq/2(Id_Command)
  "Flux_weakening "/2(Iq_ref) -> Set_Idq/3(Iq_Command), Scope1/2  "Iq_ref"
  Constant1/1 -> "Flux_weakening "/1(Enable)
  Inverse_Park_Transform/1(Alpha) -> Scope6/1, Valpha/1, Subsystem1/4(Ualpha)  "V_alpha"
  Inverse_Park_Transform/2(Beta) -> Scope6/2, Vbeta/1, Subsystem1/5(Ubeta)  "V_beta"
  Phase_CurrentABC/1 -> HF_Observer/2(Phase_CurrentABC), Clarke_Transform/1(Phase_CurrentABC)  "Phase_CurrentABC"
  Sum/1 -> Inverse_Park_Transform/1(D)
  HF_Observer/3(HFI_signal) -> Sum/2
  HF_Observer/4(speed_est) -> HFI_Speed/1
  Angle_Theta/1 -> Scope7/2, Angle_set/1(Reso_angle)  "Angle_Theta"
  Mux2/1 -> HF_Observer/1(Ialpha-beta)
  HF_Observer/5(theta_est) -> HFI_Theta/1, Scope7/1, Angle_set/2(HFI_angle)
  Merge/1 -> Scope7/3, Sine_Cosine/1(P)
  Angle_set/1(Out1) -> Merge/1
  Angle_set/2(Out2) -> Merge/2
  Subsystem1/1(Ualpha_out) -> SVPWM/1(Valpha)
  Subsystem1/2(Ubeta_out) -> SVPWM/2(Vbeta)
  HF_Observer/6(Ualpha) -> Subsystem1/2(HFI_Ualpha)
  HF_Observer/7(Ubeta) -> Subsystem1/3(HFI_Ubeta)
  HF_Observer/2(HFI_State) -> Subsystem1/1(HFI_State)
  HF_Observer/1(RUN_State) -> Angle_set/3(HFI_state), Set_Idq/1(HFI_state), RUN_State/1
  Set_Idq/1(Id) -> D_Current_PI/1(Current_Command)
  Set_Idq/2(Iq) -> Q_Current_PI/1(Current_Command)
  HF_Observer/8(IPD_Theta) -> Angle_set/4(IPD_Angle)

== system PMSM_FOC_Tractio/Motor_Control/Motor_Control_Funtion/FOC_Control_100us/Iq_selector ==
  Motor_state : Inport
  PI_IQ : Inport  Port=2
  OPL_IQ : Inport  Port=3
  If1 : If  IfExpression=u1 ==2
  Merge : Merge
  Subsystem : Subsystem
  Subsystem1 : Subsystem
  Iq_ref : Outport
  wires:
  Motor_state/1 -> If1/1
  If1/1 -> Subsystem/Action
  OPL_IQ/1 -> Subsystem/1(In1)
  PI_IQ/1 -> Subsystem1/1(In1)
  Subsystem/1(Out1) -> Merge/1
  Subsystem1/1(Out1) -> Merge/2
  Merge/1 -> Iq_ref/1
  If1/2 -> Subsystem1/Action

== system PMSM_FOC_Tractio/Motor_Control/Motor_Control_Funtion/FOC_Control_100us/MTPA ==
  Te_ref : Inport
  1-D Lookup Table4 : Lookup_n-D  NumberOfTableDimensions=1  LookupTableObject=''  BreakpointsForDimension1=single(linspace(MTPA_Te_Min,MTPA_Te_Max,length(MTPA_id_table)));  BreakpointsForDimension1FirstPoint=10  BreakpointsForDimension2FirstPoint=10  BreakpointsForDimension1Spacing=12  BreakpointsForDimension2Spacing=12  IndexSearchMethod=Evenly spaced points  Table=MTPA_id_table  InterpMethod=Flat  DiagnosticForOutOfRangeInput=Error  InternalRulePriority=Speed  RndMeth=Simplest  InputSameDT=on
  1-D Lookup Table5 : Lookup_n-D  NumberOfTableDimensions=1  LookupTableObject=''  BreakpointsForDimension1=single(linspace(MTPA_Te_Min,MTPA_Te_Max,length(MTPA_id_table)));  BreakpointsForDimension1FirstPoint=10  BreakpointsForDimension2FirstPoint=10  BreakpointsForDimension1Spacing=12  BreakpointsForDimension2Spacing=12  IndexSearchMethod=Evenly spaced points  Table=MTPA_iq_table  InterpMethod=Flat  DiagnosticForOutOfRangeInput=Error  InternalRulePriority=Speed  RndMeth=Simplest  InputSameDT=on
  Saturation : Saturate  UpperLimit=MTPA_Te_Max-0.01  LowerLimit=MTPA_Te_Min+0.01
  Saturation1 : Saturate  UpperLimit=MTPA_Te_Max-0.01  LowerLimit=MTPA_Te_Min+0.01
  Id_ref : Outport
  Iq_ref : Outport  Port=2
  wires:
  Te_ref/1 -> Saturation1/1, Saturation/1
  Saturation/1 -> 1-D Lookup Table4/1
  Saturation1/1 -> 1-D Lookup Table5/1
  1-D Lookup Table4/1 -> Id_ref/1
  1-D Lookup Table5/1 -> Iq_ref/1

== system PMSM_FOC_Tractio/Motor_Control/Motor_Control_Funtion/Angle_Speed_100us/Angle_Selector/Subsystem ==
  In1 : Inport
  Action Port : ActionPort  ActionPortLabel=if(u1 ==2)
  Out1 : Outport
  wires:
  In1/1 -> Out1/1

== system PMSM_FOC_Tractio/Motor_Control/Motor_Control_Funtion/Angle_Speed_100us/Angle_Selector/Subsystem1 ==
  In1 : Inport
  Action Port : ActionPort  ActionPortLabel=elseif(u1 ==3)
  Out1 : Outport
  wires:
  In1/1 -> Out1/1

== system PMSM_FOC_Tractio/Motor_Control/Motor_Control_Funtion/Angle_Speed_100us/Resolver_Observer/Angle_calibration ==
  Angle_input : Inport
  Angle_offset : Constant  Value=CL_Param.Angle_offset
  If Action Subsystem1 : Subsystem  TreatAsAtomicUnit=on
  If Action Subsystem2 : Subsystem  TreatAsAtomicUnit=on
  If1 : If  IfExpression=u1 > 6.283185307
  Merge1 : Merge
  Subtract1 : Sum
  Angle_output : Outport
  wires:
  Angle_input/1 -> Subtract1/1
  Merge1/1 -> Angle_output/1
  Angle_offset/1 -> Subtract1/2  "Control_ModeCommand"
  If1/1 -> If Action Subsystem2/Action
  If1/2 -> If Action Subsystem1/Action
  If Action Subsystem2/1(Out1) -> Merge1/1
  Subtract1/1 -> If Action Subsystem1/1(In1), If Action Subsystem2/1(In1), If1/1
  If Action Subsystem1/1(Out1) -> Merge1/2

== system PMSM_FOC_Tractio/Motor_Control/Motor_Control_Funtion/Angle_Speed_100us/Resolver_Observer/Resolver_Angle_cacl ==
  Sin_Cos : Inport
  2*pi : Constant  Value=2*pi  OutDataTypeStr=single  SampleTime=-1
  B : Selector  IndexMode=Zero-based  InputPortWidth=2  IndexOptions=Index vector (dialog)  Indices=0  OutputSizes=1
  C : Selector  IndexMode=Zero-based  InputPortWidth=2  IndexOptions=Index vector (dialog)  Indices=1  OutputSizes=1
  Constant : Constant  OutDataTypeStr=single  SampleTime=-1
  Discrete-Time Integrator : DiscreteIntegrator  SampleTime=-1  ICPrevOutput=DiscIntNeverNeededParam  ICPrevScaledInput=DiscIntNeverNeededParam
  Gain : Gain  Gain=15/(2*pi)
  LPF : DiscreteFilter  Numerator=[0 0.04]  Denominator=[1 -0.96]
  Math Function : Math  Operator=mod  SaturateOnIntegerOverflow=on
  PID Controller : simulink/Continuous/PID Controller  Controller=PI  Form=Parallel  TimeDomain=Discrete-time  SampleTime=-1  IntegratorMethod=Forward Euler  FilterMethod=Forward Euler  ControllerParametersSource=internal  P=141  I=10000  D=0  UseFilter=off  N=100  TunerSelectOption=Transfer Function Based (PID Tuner App)  InitialConditionSource=internal  InitialConditionForIntegrator=0  InitialConditionForFilter=0  DifferentiatorICPrevScaledInput=0  ExternalReset=none  TrackingMode=off  Kt=1  LimitOutput=off  UpperSaturationLimit=inf  LowerSaturationLimit=-inf  LinearizeAsGain=on  AntiWindupMode=none  Kb=1  POutMin=[]  POutMax=[]  IOutMin=[]  IOutMax=[]  DOutMin=[]  DOutMax=[]  NOutMin=[]  NOutMax=[]  SumOutMin=[]  SumOutMax=[]  SaturationOutMin=[]  SaturationOutMax=[]  PParamMin=[]  PParamMax=[]  IParamMin=[]  IParamMax=[]  DParamMin=[]  DParamMax=[]  NParamMin=[]  NParamMax=[]  KbParamMin=[]  KbParamMax=[]  KtParamMin=[]  KtParamMax=[]  KbOutMin=[]  KbOutMax=[]  KtOutMin=[]  KtOutMax=[]  IntegratorOutMin=[]  IntegratorOutMax=[]  FilterOutMin=[]  FilterOutMax=[]  SumI1OutMin=[]  SumI1OutMax=[]  SumI2OutMin=[]  SumI2OutMax=[]  SumI3OutMin=[]  SumI3OutMax=[]  SumI4OutMin=[]  SumI4OutMax=[]  SumDOutMin=[]  SumDOutMax=[]  DifferentiatorOutMin=[]  DifferentiatorOutMax=[]  FilterDiffOutCoefMin=[]  FilterDiffOutCoefMax=[]  ReciprocalOutMin=[]  ReciprocalOutMax=[]  SumDenOutMin=[]  SumDenOutMax=[]  SumNumOutMin=[]  SumNumOutMax=[]  DivideOutMin=[]  DivideOutMax=[]  IntegratorContinuousStateAttributes=''  IntegratorStateMustResolveToSignalObject=off  IntegratorRTWStateStorageClass=Auto  FilterContinuousStateAttributes=''  FilterStateMustResolveToSignalObject=off  FilterRTWStateStorageClass=Auto  ParallelPVariant=InternalParameters  IdealPVariant=Disabled  IVariant=InternalParameters  DVariant=Disabled  IntegratorVariant=Discrete  SatVariant=Disabled  AWVariant=Passthrough  PCopyVariant=Disabled  TRVariant=Disabled  FdbkBlocksVariant=Forward  IdealPFdbkVariant=Disabled  SatFdbkVariant=Disabled  DerivativeFilterVariant=Disabled  NVariant=Disabled  NCopyVariant=Disabled_SignalSpec  FilterICVariant=Disabled  IntegratorICVariant=InternalICs  ExternalResetVariant=Disabled  TRSumVariant=Passthrough  SumFdbkVariant=Disabled  SumVariant=Sum_PI
  Product : Product  OutDataTypeStr=single
  Product{1..4} (4 alike) : Product
  Scope : Scope  NumInputPorts=2
  Scope{1,3..4,6..7} (5 alike) : Scope
  Scope2 : Scope  NumInputPorts=2
  Scope5 : Scope  NumInputPorts=2
  Sine_Cosine : Subsystem  TreatAsAtomicUnit=on
      settings: RTWSystemCode=Nonreusable function  RTWFcnNameOpts=Use subsystem name
  Sum1 : Sum  Inputs=-+
  Unit Delay4 : UnitDelay  SampleTime=-1  HasFrameUpgradeWarning=on
  constant : Constant  OutDataTypeStr=single
  "pole pairs " : Gain  OutDataTypeStr=single
  Velocity : Outport  VectorParamsAs1DForOutWhenUnconnected=off
  Angle : Outport  Port=2  VectorParamsAs1DForOutWhenUnconnected=off
  wires:
  Product2/1 -> Scope2/2, Product4/1
  Product4/1 -> Scope/2, Sum1/2
  Sin_Cos/1 -> C/1, B/1
  Unit Delay4/1 -> Product/2
  Sum1/1 -> PID Controller/1
  Product3/1 -> Scope/1, Sum1/1
  Constant/1 -> Product/1
  constant/1 -> Product2/1, Product1/1
  Product/1 -> Sine_Cosine/1(P)
  Sine_Cosine/1(Sin) -> Product1/2
  Product1/1 -> Scope2/1, Product3/2
  Math Function/1 -> Unit Delay4/1, Angle/1, Scope4/1  "Angle_Theta"
  Gain/1 -> LPF/1, Scope3/1  "Speed_RPM"
  Discrete-Time Integrator/1 -> Scope6/1, "pole pairs "/1
  "pole pairs "/1 -> Math Function/1
  PID Controller/1 -> Discrete-Time Integrator/1, Gain/1
  2*pi/1 -> Math Function/2
  B/1 -> Scope1/1, Product3/1, Scope5/2, Scope5/1  "Vx"
  C/1 -> Product4/2, Scope7/1  "Vy"
  LPF/1 -> Velocity/1
  Sine_Cosine/2(Cos) -> Product2/2

== system PMSM_FOC_Tractio/Motor_Control/Motor_Control_Funtion/Angle_Speed_100us/SMO/Angle_calibration ==
  Angle_input : Inport
  Angle_offset : Constant  Value=SMO.Angle_offset
  If Action Subsystem1 : Subsystem  TreatAsAtomicUnit=on
  If Action Subsystem2 : Subsystem  TreatAsAtomicUnit=on
  If Action Subsystem3 : Subsystem  TreatAsAtomicUnit=on
  If1 : If  IfExpression=u1 > 6.283185307  ElseIfExpressions=u1<0
  Merge1 : Merge  Inputs=3
  Subtract1 : Sum
  Angle_output : Outport
  wires:
  Angle_input/1 -> Subtract1/1
  Angle_offset/1 -> Subtract1/2  "Control_ModeCommand"
  If1/1 -> If Action Subsystem2/Action
  If1/3 -> If Action Subsystem1/Action
  If Action Subsystem2/1(Out1) -> Merge1/1
  Subtract1/1 -> If Action Subsystem3/1(In1), If Action Subsystem1/1(In1), If Action Subsystem2/1(In1), If1/1
  If Action Subsystem1/1(Out1) -> Merge1/3
  If Action Subsystem3/1(Out1) -> Merge1/2
  If1/2 -> If Action Subsystem3/Action
  Merge1/1 -> Angle_output/1

== system PMSM_FOC_Tractio/Motor_Control/Motor_Control_Funtion/Angle_Speed_100us/SMO/Delta_theta ==
  Est_theta : Inport
  Ealpha_est : Inport  Port=2
  Ebeta_est : Inport  Port=3
  Add : Sum
  Add1 : Sum
  Divide : Product  Inputs=*/
  Gain : Gain  Gain=-1
  Math Function : Math  Operator=magnitude^2  SignedPower=off  SaturateOnIntegerOverflow=on
  Math Function1 : Math  Operator=magnitude^2  SignedPower=off  SaturateOnIntegerOverflow=on
  Product : Product
  Product1 : Product
  Saturation : Saturate  UpperLimit=inf  LowerLimit=4.0
  Sine_Cosine : Subsystem  TreatAsAtomicUnit=on
      settings: RTWSystemCode=Nonreusable function  RTWFcnNameOpts=Use subsystem name
  Sqrt : Sqrt  SaturateOnIntegerOverflow=on
  delta_theta : Outport
  unit : Outport  Port=2
  wires:
  Est_theta/1 -> Sine_Cosine/1(P)
  Ealpha_est/1 -> Math Function/1, Product/2
  Sine_Cosine/1(Sin) -> Product1/1
  Ebeta_est/1 -> Math Function1/1, Product1/2
  Product/1 -> Add/1
  Product1/1 -> Add/2
  Add/1 -> Gain/1
  Math Function/1 -> Add1/1
  Math Function1/1 -> Add1/2
  Add1/1 -> Sqrt/1
  Sqrt/1 -> Saturation/1
  Gain/1 -> Divide/1
  Saturation/1 -> unit/1, Divide/2
  Divide/1 -> delta_theta/1
  Sine_Cosine/2(Cos) -> Product/1

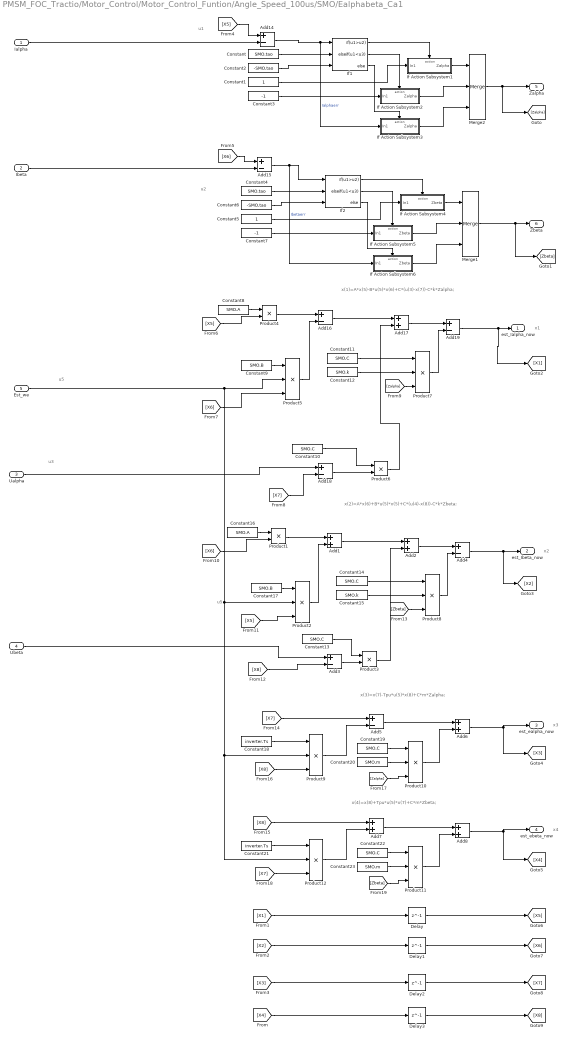
== system PMSM_FOC_Tractio/Motor_Control/Motor_Control_Funtion/Angle_Speed_100us/SMO/Ealphabeta_Ca1 ==
  note: x(4)=x(8)+Tpu*u(5)*x(7)+C*m*Zbeta;
  note: x(3)=x(7)-Tpu*u(5)*x(8)+C*m*Zalpha;
  note: x(2)=A*x(6)+B*u(5)*x(5)+C*(u(4)-x(8))-C*k*Zbeta;
  note: x(1)=A*x(5)-B*u(5)*x(6)+C*(u(3)-x(7))-C*k*Zalpha;
  note: x1
  note: u1
  note: u3
  note: u5
  note: u2
  note: u5
  note: x2
  note: x3
  note: x4
  Ialpha : Inport
  Ibeta : Inport  Port=2
  Ualpha : Inport  Port=3
  Ubeta : Inport  Port=4
  Est_we : Inport  Port=5
  Add{1..2,6..8,17} (6 alike) : Sum
  Add{3..5,14..16,18..19} (8 alike) : Sum  Inputs=+-
  Constant : Constant  Value=SMO.tao  OutDataTypeStr=single
  Constant1 : Constant  OutDataTypeStr=single
  Constant10 : Constant  Value=SMO.C  OutDataTypeStr=single
  Constant11 : Constant  Value=SMO.C  OutDataTypeStr=single
  Constant12 : Constant  Value=SMO.k  OutDataTypeStr=single
  Constant{13..14,19,22} (4 alike) : Constant  Value=SMO.C
  Constant15 : Constant  Value=SMO.k
  Constant16 : Constant  Value=SMO.A  OutDataTypeStr=single
  Constant17 : Constant  Value=SMO.B
  Constant18 : Constant  Value=inverter.Ts  OutDataTypeStr=single
  Constant2 : Constant  Value=-SMO.tao  OutDataTypeStr=single
  Constant20 : Constant  Value=SMO.m
  Constant21 : Constant  Value=inverter.Ts  OutDataTypeStr=single
  Constant23 : Constant  Value=SMO.m
  Constant3 : Constant  Value=-1  OutDataTypeStr=single
  Constant4 : Constant  Value=SMO.tao
  Constant5 : Constant  OutDataTypeStr=single
  Constant6 : Constant  Value=-SMO.tao
  Constant7 : Constant  Value=-1  OutDataTypeStr=single
  Constant8 : Constant  Value=SMO.A  OutDataTypeStr=single
  Constant9 : Constant  Value=SMO.B
  Delay{,1..3} (4 alike) : Delay  DelayLength=1  InitialCondition=0
  If Action Subsystem1 : Subsystem  TreatAsAtomicUnit=on
  If Action Subsystem2 : Subsystem  TreatAsAtomicUnit=on
  If Action Subsystem3 : Subsystem  TreatAsAtomicUnit=on
  If Action Subsystem4 : Subsystem  TreatAsAtomicUnit=on
  If Action Subsystem5 : Subsystem  TreatAsAtomicUnit=on
  If Action Subsystem6 : Subsystem  TreatAsAtomicUnit=on
  If1 : If  NumInputs=3  IfExpression=u1>u2  ElseIfExpressions=u1<u3
  If2 : If  NumInputs=3  IfExpression=u1>u2  ElseIfExpressions=u1<u3
  Merge1 : Merge  Inputs=3
  Merge2 : Merge  Inputs=3
  Product{1,3..4,6} (4 alike) : Product
  Product{2,5,7..12} (8 alike) : Product  Inputs=3
  est_Ialpha_now : Outport
  est_Ibeta_now : Outport  Port=2
  est_ealpha_now : Outport  Port=3
  est_ebeta_now : Outport  Port=4
  Zalpha : Outport  Port=5
  Zbeta : Outport  Port=6
  wires:
  Ialpha/1 -> Add14/2
  Add14/1 -> If Action Subsystem3/1(In1), If1/1  "Ialphaerr"
  Constant/1 -> If1/2
  If1/1 -> If Action Subsystem1/Action
  Constant1/1 -> If Action Subsystem1/1(In1)
  Constant3/1 -> If Action Subsystem2/1(In1)
  Constant2/1 -> If1/3
  If1/2 -> If Action Subsystem2/Action
  If1/3 -> If Action Subsystem3/Action
  If Action Subsystem1/1(Zalpha) -> Merge2/1
  If Action Subsystem2/1(Zalpha) -> Merge2/2
  If Action Subsystem3/1(Zalpha) -> Merge2/3
  Ibeta/1 -> Add15/2
  If2/1 -> If Action Subsystem4/Action
  If2/3 -> If Action Subsystem6/Action
  If Action Subsystem4/1(Zbeta) -> Merge1/1
  Constant5/1 -> If Action Subsystem4/1(In1)
  If2/2 -> If Action Subsystem5/Action
  Constant6/1 -> If2/3
  If Action Subsystem6/1(Zbeta) -> Merge1/3
  Constant7/1 -> If Action Subsystem5/1(In1)
  If Action Subsystem5/1(Zbeta) -> Merge1/2
  Add15/1 -> If2/1, If Action Subsystem6/1(In1)  "Ibetaerr"
  Constant4/1 -> If2/2
  Constant8/1 -> Product4/1
  Add19/1 -> [X1], est_Ialpha_now/1
  Product4/1 -> Add16/1
  Constant9/1 -> Product5/1
  Product5/1 -> Add16/2
  Add16/1 -> Add17/1
  Ualpha/1 -> Add18/1
  Add18/1 -> Product6/2
  Constant10/1 -> Product6/1
  Product6/1 -> Add17/2
  Add17/1 -> Add19/1
  Product7/1 -> Add19/2
  Constant11/1 -> Product7/1
  Constant12/1 -> Product7/2
  Product3/1 -> Add2/2
  Product8/1 -> Add4/2
  Constant15/1 -> Product8/2
  Constant16/1 -> Product1/1
  Add3/1 -> Product3/2
  Product2/1 -> Add1/2
  Add4/1 -> [X2], est_Ibeta_now/1
  Constant14/1 -> Product8/1
  Add1/1 -> Add2/1
  Constant13/1 -> Product3/1
  Ubeta/1 -> Add3/1
  Constant17/1 -> Product2/1
  Add2/1 -> Add4/1
  Product1/1 -> Add1/1
  Add6/1 -> est_ealpha_now/1, [X3]
  Constant18/1 -> Product9/1
  Product9/1 -> Add5/2
  Add5/1 -> Add6/1
  Constant19/1 -> Product10/1
  Constant20/1 -> Product10/2
  Product10/1 -> Add6/2
  Merge1/1 -> [Zbeta], Zbeta/1
  Constant21/1 -> Product12/1
  Constant22/1 -> Product11/1
  Est_we/1 -> Product12/2, Product9/2, Product2/2, Product5/2
  Product12/1 -> Add7/2
  Constant23/1 -> Product11/2
  Product11/1 -> Add8/2
  Add7/1 -> Add8/1
  Add8/1 -> [X4], est_ebeta_now/1
  Merge2/1 -> [Zalpha], Zalpha/1
  [X1] -> Delay/1
  [X2] -> Delay1/1
  [X3] -> Delay2/1
  [X4] -> Delay3/1
  Delay/1 -> [X5]
  Delay1/1 -> [X6]
  Delay2/1 -> [X7]
  Delay3/1 -> [X8]
  [X5] -> Add14/1
  [X6] -> Add15/1
  [X5] -> Product4/2
  [X6] -> Product5/3
  [X7] -> Add18/2
  [Zalpha] -> Product7/3
  [X6] -> Product1/2
  [X5] -> Product2/3
  [X8] -> Add3/2
  [Zbeta] -> Product8/3
  [X7] -> Add5/1
  [X8] -> Add7/1
  [X8] -> Product9/3
  [Zalpha] -> Product10/3
  [X7] -> Product12/3
  [Zbeta] -> Product11/3

== system PMSM_FOC_Tractio/Motor_Control/Motor_Control_Funtion/Angle_Speed_100us/SMO/PLL_PI ==
  in : Inport
  Add : Sum
  Discrete-Time Integrator : DiscreteIntegrator  SampleTime=Ts  ICPrevOutput=DiscIntNeverNeededParam  ICPrevScaledInput=DiscIntNeverNeededParam
  Gain2 : Gain  Gain=kp
  Gain3 : Gain  Gain=ki
  Saturation : Saturate  UpperLimit=inf  LowerLimit=-inf
  Scope : Scope  NumInputPorts=3
  Out : Outport
  wires:
  Gain2/1 -> Scope/1, Add/1
  Gain3/1 -> Discrete-Time Integrator/1
  Discrete-Time Integrator/1 -> Scope/2, Add/2
  in/1 -> Gain3/1, Gain2/1
  Add/1 -> Saturation/1
  Saturation/1 -> Scope/3, Out/1

== system PMSM_FOC_Tractio/Motor_Control/Motor_Control_Funtion/Angle_Speed_100us/Speed_Resolver/Speed_cacl ==
  position : Inport  OutMin=-4*pi  OutMax=4*pi
      settings: AttributesFormatString="------------------\\nMin =  %<OutMin>\\nMax =  %<OutMax>"
  Convert_to_Uint32 : DataTypeConversion  OutDataTypeStr=int32  RndMeth=Simplest
  Difference_Wrap : Sum  Inputs=+-  AccumDataTypeStr=int32  OutDataTypeStr=int32
  Difference_to_Single : DataTypeConversion  OutDataTypeStr=single
  LPF : DiscreteFilter  Numerator=[0 0.5]  Denominator=[1 -0.5]
  Position_Delay : Delay  DelayLength=1
  RPM_Gain : Gain  Gain=60/(2*pi*pmsm.PolePairs)  ParamDataTypeStr=single  OutDataTypeStr=single
      settings: AttributesFormatString=---------------------------------\n%<Gain>
  Scale_Input : Gain  Gain=((2^31) - 1)/(4*pi)  ParamDataTypeStr=single  OutDataTypeStr=single
      settings: AttributesFormatString=---------------------------------\n%<Gain>
  Scale_Output : Gain  Gain=pi/(2^31 -1)/(inverter.Ts)  ParamDataTypeStr=single  OutDataTypeStr=single
      settings: AttributesFormatString=---------------------------------\n%<Gain>
  Scope1 : Scope  NumInputPorts=2
  Scope7 : Scope  NumInputPorts=2
  Wrap_To_Pi : Gain  Gain=4  RndMeth=Simplest  OutDataTypeStr=Inherit: Same as input  ParamDataTypeStr=Inherit: Same as input
  Speed_RPM : Outport  VectorParamsAs1DForOutWhenUnconnected=off
  wires:
  position/1 -> Scale_Input/1  "position"
  Scale_Input/1 -> Convert_to_Uint32/1
  Difference_to_Single/1 -> Scope7/1, Scale_Output/1
  Wrap_To_Pi/1 -> Difference_Wrap/1, Position_Delay/1
  Scale_Output/1 -> RPM_Gain/1  "We"
  Position_Delay/1 -> Difference_Wrap/2
  Convert_to_Uint32/1 -> Wrap_To_Pi/1
  Difference_Wrap/1 -> Difference_to_Single/1
  RPM_Gain/1 -> Scope7/2, Scope1/2, LPF/1  "Speed_RPM"
  LPF/1 -> Scope1/1, Speed_RPM/1  "Speed_RPM_Filtered"

== system PMSM_FOC_Tractio/Motor_Control/Motor_Control_Funtion/Control_Command_2ms/Speed_PI/Speed_PI ==
  PI_input : Inport
  HFI_State : Inport  Port=2
  HFI_Enalble : Constant  Value=HFI.Func_Enable  OutDataTypeStr=uint8
  If1 : If  NumInputs=2  IfExpression=(u1==3)&(u2==1)  ElseIfExpressions=(u2==0)  ShowElse=off
  Merge : Merge
  Speed_Control : Subsystem
  Speed_Control1 : Subsystem
  PI_out : Outport  VectorParamsAs1DForOutWhenUnconnected=off
  wires:
  PI_input/1 -> Speed_Control1/1(Err), Speed_Control/1(Err)
  HFI_State/1 -> If1/1
  If1/1 -> Speed_Control/Action
  HFI_Enalble/1 -> If1/2
  If1/2 -> Speed_Control1/Action
  Merge/1 -> PI_out/1
  Speed_Control/1(PI_Out) -> Merge/1
  Speed_Control1/1(PI_Out) -> Merge/2

== system PMSM_FOC_Tractio/Motor_Control/Motor_Control_Funtion/FOC_Control_100us/FOC/Angle_set ==
  Reso_angle : Inport
  HFI_angle : Inport  Port=2
  HFI_state : Inport  Port=3
  IPD_Angle : Inport  Port=4
  HFI_AngleEnable : Constant  Value=HFI.Angle_Enable  OutDataTypeStr=uint8
  If1 : If  IfExpression=u1 ==1
  Subsystem : Subsystem
  Subsystem1 : Subsystem
  Out1 : Outport
  Out2 : Outport  Port=2
  wires:
  HFI_AngleEnable/1 -> If1/1
  If1/1 -> Subsystem/Action
  HFI_angle/1 -> Subsystem/2(HFI_angle)
  If1/2 -> Subsystem1/Action
  Reso_angle/1 -> Subsystem1/1(Reso_angle)
  Subsystem/1(Out1) -> Out1/1
  Subsystem1/1(Out1) -> Out2/1
  HFI_state/1 -> Subsystem/1(HFI_state)
  IPD_Angle/1 -> Subsystem/3(IPD_Angle)

== system PMSM_FOC_Tractio/Motor_Control/Motor_Control_Funtion/FOC_Control_100us/FOC/Clarke_Transform ==
  Phase_CurrentABC : Inport  PortDimensions=3
  Clark1 : Subsystem  TreatAsAtomicUnit=on
  Scope : Scope  NumInputPorts=2
  IAlpha : Outport  VectorParamsAs1DForOutWhenUnconnected=off
  IBeta : Outport  Port=2  VectorParamsAs1DForOutWhenUnconnected=off
  wires:
  Clark1/1(Ialpha) -> IAlpha/1, Scope/1
  Clark1/2(Ibeta) -> IBeta/1, Scope/2
  Phase_CurrentABC/1 -> Clark1/1(Iabc)

== system PMSM_FOC_Tractio/Motor_Control/Motor_Control_Funtion/FOC_Control_100us/FOC/D_Current_PI ==
  Current_Command : Inport
  Current_Measured : Inport  Port=2
  Add2 : Sum  Inputs=|+-
  ID_Control : Subsystem
  Vd_voltage : Outport  VectorParamsAs1DForOutWhenUnconnected=off
  wires:
  Current_Command/1 -> Add2/1
  Current_Measured/1 -> Add2/2
  Add2/1 -> ID_Control/1(Err)  "currentControlError"
  ID_Control/1(PI_Out) -> Vd_voltage/1
